simulink subsystem "MultibodySuspensionSSC"  (R2024a)
settings: Solver=VariableStepAuto  StartTime=0.0  StopTime=10.0  RelTol=1e-3
undefined symbols (not defined in the file): EnvGrvty, FrntRef, LAc, LAf, LAr, PlntVehDstCGFrntAxl, PlntVehDstCGRearAxl, PlntVehMass, PlntVehMultiBody, PlntVehMultiBodyGeom, RearRef, StrRodFL, StrRodFR, StrRodRL, StrRodRR, UAc, UAf, UAr, WheelFL, WheelFR, WheelRL, WheelRR, X, Y, Z
libraries: sm_lib x450, fl_lib x96, nesl_utility x64, sdl_lib x8
(part 10 of 17)

== system MultibodySuspensionSSC/SuspF/Linkage/Linkage R/DoubleWishbone/Upright ==
  note: Axle length still distance from
      | Wheel Center to Upright midpoint
  Axle : sm_lib/Body Elements/Cylindrical Solid  CylinderRadius=radius_stub_axle  CylinderRadiusUnits=m  CylinderLength=len_axle*2  CylinderLengthUnits=m  ExportEntireGeometry=off  InertiaType=PointMass  BasedOnType=Mass  Density=7000  DensityUnits=kg/m^3  Mass=0  MassUnits=kg  CenterOfMass=[0 0 0]  CenterOfMassUnits=m  MomentsOfInertia=[1 1 1]  MomentsOfInertiaUnits=kg*m^2  ProductsOfInertia=[0 0 0]  ProductsOfInertiaUnits=kg*m^2  GraphicType=FromGeometry  MarkerShape=Sphere  MarkerSize=10  GraphicVisPropType=SimpleVisualProperties  GraphicDiffuseColor=clr_stub_axle  GraphicOpacity=opc_stub_axle  GraphicSpecularColor=[0.5 0.5 0.5 1.0]  GraphicAmbientColor=[0.15 0.15 0.15 1.0]  GraphicEmissiveColor=[0.0 0.0 0.0 1.0]  GraphicShininess=75  DoExposeReferenceFrame=on  SerializedFrames=<Frames/>
      settings: LibrarySourceBlock=sm_car_4post_lib/Suspension and Steering/Linkage/Linkage R/DoubleWishbone/Upright/Axle
  Inertia CG : sm_lib/Body Elements/Inertia  InertiaType=PointMass  Mass=upr_mass  MassUnits=kg  CenterOfMass=[0 0 0]  CenterOfMassUnits=m  MomentsOfInertia=[1 1 1]  MomentsOfInertiaUnits=kg*m^2  ProductsOfInertia=[0 0 0]  ProductsOfInertiaUnits=kg*m^2  GraphicType=Marker  MarkerShape=Inertia  MarkerSize=20  GraphicVisPropType=SimpleVisualProperties  GraphicDiffuseColor=[0.5 0.5 0.5]  GraphicOpacity=0  GraphicSpecularColor=[0.5 0.5 0.5 1.0]  GraphicAmbientColor=[0.15 0.15 0.15 1.0]  GraphicEmissiveColor=[0.0 0.0 0.0 1.0]  GraphicShininess=75
      settings: LibrarySourceBlock=|
      | sm_car_4post_lib/Suspension and Steering/Linkage/Linkage R/DoubleWishbone/Upright/Inertia
      | CG
  Steering Arm : Subsystem  mask{hp_b=(hp_la_out+(35/300)*(hp_ua_out-hp_la_out)).*rhs_hp, hp_f=hp_upr_rod.*rhs_hp, Mass=0, clr_solid=clr_upr, opc_solid=opc_upr, rad_solid=radius_upr}
      mask prompts: hp_b "Hardpoint at B [xyz] (m)"; hp_f "Hardpoint at F [xyz] (m)"; Mass "Mass (kg)"; clr_solid "Color [RGB]"; opc_solid "Opacity (0-1)"; rad_solid "Radius (m)"
      settings: LibrarySourceBlock=sm_car_4post_lib/Suspension and Steering/Linkage/Linkage R/DoubleWishbone/Upright/Steering Arm
      mask TypeOptions Mass: Solid/Mass
      mask TypeOptions clr_solid: Solid/GraphicDiffuseColor
      mask TypeOptions opc_solid: Solid/GraphicOpacity
      mask TypeOptions rad_solid: Solid/CylinderRadius
      mask DialogControl cont_vis Prompt: Visualization
  Transform Align for Universal Joint : Subsystem  mask(Transform Align Axis Two Points){hp_b=(hp_la_out+0.5*(hp_ua_out-hp_la_out)).*rhs_hp, hp_t=hp_upr_rod.*rhs_hp, popup_f_axis=+Z}
      mask prompts: hp_b "Location of B [xyz] (m)"; hp_t "Target for Frame Axis [xyz] (m)"; popup_f_axis "Axis of F Frame to Aim at Target"
      mask help: Transforms a frame to aim a selected axis at a target point. Both points must be defined relative to the same reference frame.
      mask init: same as MultibodySuspensionSSC/SuspF/Linkage/Linkage L/DoubleWishbone/Hardpoints/Transform Align LAf LAr
      settings: LibrarySourceBlock=|
      | sm_car_4post_lib/Suspension and Steering/Linkage/Linkage R/DoubleWishbone/Upright/Transform
      | Align for
      | Universal
      | Joint
      mask TypeOptions popup_f_axis: +X | +Y | +Z | -X | -Y | -Z
  Transform Toe Camber : sm_lib/Frames and Transforms/Rigid Transform  RotationMethod=RotationSequence  FollAlignAxisA=+X  BaseAlignAxisA=+Y  FollAlignAxisB=+Y  BaseAlignAxisB=+Z  RotationStandardAxis=+Z  RotationAngle=0.0  RotationAngleUnits=deg  RotationArbitraryAxis=[0 0 1]  RotationSequenceAxes=FollowerAxes  RotationSequence=YXY  RotationSequenceAngles=[atoe -acamber 0].*rhs_upr  RotationSequenceAnglesUnits=deg  RotationMatrix=[1 0 0; 0 1 0; 0 0 1]  Quaternion=[1 0 0 0]  TranslationMethod=None  TranslationCartesianOffset=[0 0 0]  TranslationCartesianOffsetUnits=m  TranslationStandardAxis=+Z  TranslationStandardOffset=0  TranslationStandardOffsetUnits=m  TranslationROffset=0  TranslationROffsetUnits=m  TranslationThetaOffset=0  TranslationThetaOffsetUnits=deg  TranslationZOffset=0  TranslationZOffsetUnits=m
      settings: LibrarySourceBlock=|
      | sm_car_4post_lib/Suspension and Steering/Linkage/Linkage R/DoubleWishbone/Upright/Transform
      | Toe Camber
  Transform Upright CG : sm_lib/Frames and Transforms/Rigid Transform  RotationMethod=None  FollAlignAxisA=+X  BaseAlignAxisA=+Y  FollAlignAxisB=+Y  BaseAlignAxisB=+Z  RotationStandardAxis=+Z  RotationAngle=0.0  RotationAngleUnits=deg  RotationArbitraryAxis=[0 0 1]  RotationSequenceAxes=FollowerAxes  RotationSequence=XYX  RotationSequenceAngles=[0 0 0]  RotationSequenceAnglesUnits=deg  RotationMatrix=[1 0 0; 0 1 0; 0 0 1]  Quaternion=[1 0 0 0]  TranslationMethod=Cartesian  TranslationCartesianOffset=(hp_upr_cg-hp_la_out) .* [1, rhs_upr, 1]  TranslationCartesianOffsetUnits=m  TranslationStandardAxis=+Z  TranslationStandardOffset=0  TranslationStandardOffsetUnits=m  TranslationROffset=0  TranslationROffsetUnits=m  TranslationThetaOffset=0  TranslationThetaOffsetUnits=deg  TranslationZOffset=0  TranslationZOffsetUnits=m
      settings: LibrarySourceBlock=|
      | sm_car_4post_lib/Suspension and Steering/Linkage/Linkage R/DoubleWishbone/Upright/Transform
      | Upright CG
  Transform Upright Ctr : sm_lib/Frames and Transforms/Rigid Transform  RotationMethod=None  FollAlignAxisA=+X  BaseAlignAxisA=+Y  FollAlignAxisB=+Y  BaseAlignAxisB=+Z  RotationStandardAxis=+Z  RotationAngle=0.0  RotationAngleUnits=deg  RotationArbitraryAxis=[0 0 1]  RotationSequenceAxes=FollowerAxes  RotationSequence=XYX  RotationSequenceAngles=[0 0 0]  RotationSequenceAnglesUnits=deg  RotationMatrix=[1 0 0; 0 1 0; 0 0 1]  Quaternion=[1 0 0 0]  TranslationMethod=Cartesian  TranslationCartesianOffset=(35/300)*(hp_ua_out-hp_la_out).*rhs_hp  TranslationCartesianOffsetUnits=m  TranslationStandardAxis=+Z  TranslationStandardOffset=0  TranslationStandardOffsetUnits=m  TranslationROffset=0  TranslationROffsetUnits=m  TranslationThetaOffset=0  TranslationThetaOffsetUnits=deg  TranslationZOffset=0  TranslationZOffsetUnits=m
      settings: LibrarySourceBlock=|
      | sm_car_4post_lib/Suspension and Steering/Linkage/Linkage R/DoubleWishbone/Upright/Transform
      | Upright Ctr
  Transform Whl Ctr : sm_lib/Frames and Transforms/Rigid Transform  RotationMethod=AlignedAxes  FollAlignAxisA=+Z  BaseAlignAxisA=+Y  FollAlignAxisB=+X  BaseAlignAxisB=+X  RotationStandardAxis=+Z  RotationAngle=0.0  RotationAngleUnits=deg  RotationArbitraryAxis=[0 0 1]  RotationSequenceAxes=FollowerAxes  RotationSequence=XYX  RotationSequenceAngles=[0 0 0]  RotationSequenceAnglesUnits=deg  RotationMatrix=[1 0 0; 0 1 0; 0 0 1]  Quaternion=[1 0 0 0]  TranslationMethod=Cartesian  TranslationCartesianOffset=(hp_upr_wc-hp_la_out) .* rhs_hp  TranslationCartesianOffsetUnits=m  TranslationStandardAxis=+Z  TranslationStandardOffset=0  TranslationStandardOffsetUnits=m  TranslationROffset=0  TranslationROffsetUnits=m  TranslationThetaOffset=0  TranslationThetaOffsetUnits=deg  TranslationZOffset=0  TranslationZOffsetUnits=m
      settings: LibrarySourceBlock=|
      | sm_car_4post_lib/Suspension and Steering/Linkage/Linkage R/DoubleWishbone/Upright/Transform
      | Whl Ctr
  Upright : Subsystem  mask{hp_b=hp_la_out.*rhs_hp, hp_f=hp_ua_out.*rhs_hp, Mass=0, clr_solid=clr_upr, opc_solid=opc_upr, rad_solid=radius_upr}
      mask prompts: hp_b "Hardpoint at B [xyz] (m)"; hp_f "Hardpoint at F [xyz] (m)"; Mass "Mass (kg)"; clr_solid "Color [RGB]"; opc_solid "Opacity (0-1)"; rad_solid "Radius (m)"
      settings: LibrarySourceBlock=sm_car_4post_lib/Suspension and Steering/Linkage/Linkage R/DoubleWishbone/Upright/Upright
      mask TypeOptions Mass: Solid/Mass
      mask TypeOptions clr_solid: Solid/GraphicDiffuseColor
      mask TypeOptions opc_solid: Solid/GraphicOpacity
      mask TypeOptions rad_solid: Solid/CylinderRadius
      mask DialogControl cont_vis Prompt: Visualization
  Vis Upright LA : sm_lib/Body Elements/Spherical Solid  SphereRadius=size_conn_upr  SphereRadiusUnits=m  ExportEntireGeometry=off  InertiaType=PointMass  BasedOnType=Density  Density=0  DensityUnits=kg/m^3  Mass=0  MassUnits=kg  CenterOfMass=[0 0 0]  CenterOfMassUnits=m  MomentsOfInertia=[1 1 1]  MomentsOfInertiaUnits=kg*m^2  ProductsOfInertia=[0 0 0]  ProductsOfInertiaUnits=kg*m^2  GraphicType=FromGeometry  MarkerShape=Sphere  MarkerSize=10  GraphicVisPropType=SimpleVisualProperties  GraphicDiffuseColor=clr_conn_upr  GraphicOpacity=opc_conn_upr  GraphicSpecularColor=[0.5 0.5 0.5 1.0]  GraphicAmbientColor=[0.15 0.15 0.15 1.0]  GraphicEmissiveColor=[0.0 0.0 0.0 1.0]  GraphicShininess=75  DoExposeReferenceFrame=on  SerializedFrames=<Frames/>
      settings: LibrarySourceBlock=sm_car_4post_lib/Suspension and Steering/Linkage/Linkage R/DoubleWishbone/Upright/Vis Upright LA
  Vis Upright UA : sm_lib/Body Elements/Spherical Solid  SphereRadius=size_conn_upr  SphereRadiusUnits=m  ExportEntireGeometry=off  InertiaType=PointMass  BasedOnType=Density  Density=0  DensityUnits=kg/m^3  Mass=0  MassUnits=kg  CenterOfMass=[0 0 0]  CenterOfMassUnits=m  MomentsOfInertia=[1 1 1]  MomentsOfInertiaUnits=kg*m^2  ProductsOfInertia=[0 0 0]  ProductsOfInertiaUnits=kg*m^2  GraphicType=FromGeometry  MarkerShape=Sphere  MarkerSize=10  GraphicVisPropType=SimpleVisualProperties  GraphicDiffuseColor=clr_conn_upr  GraphicOpacity=opc_conn_upr  GraphicSpecularColor=[0.5 0.5 0.5 1.0]  GraphicAmbientColor=[0.15 0.15 0.15 1.0]  GraphicEmissiveColor=[0.0 0.0 0.0 1.0]  GraphicShininess=75  DoExposeReferenceFrame=on  SerializedFrames=<Frames/>
      settings: LibrarySourceBlock=sm_car_4post_lib/Suspension and Steering/Linkage/Linkage R/DoubleWishbone/Upright/Vis Upright UA
  Vis Wheel Center : sm_lib/Body Elements/Spherical Solid  SphereRadius=size_conn_upr  SphereRadiusUnits=m  ExportEntireGeometry=off  InertiaType=PointMass  BasedOnType=Density  Density=0  DensityUnits=kg/m^3  Mass=0  MassUnits=kg  CenterOfMass=[0 0 0]  CenterOfMassUnits=m  MomentsOfInertia=[1 1 1]  MomentsOfInertiaUnits=kg*m^2  ProductsOfInertia=[0 0 0]  ProductsOfInertiaUnits=kg*m^2  GraphicType=FromGeometry  MarkerShape=Sphere  MarkerSize=10  GraphicVisPropType=SimpleVisualProperties  GraphicDiffuseColor=clr_conn_upr  GraphicOpacity=opc_conn_upr  GraphicSpecularColor=[0.5 0.5 0.5 1.0]  GraphicAmbientColor=[0.15 0.15 0.15 1.0]  GraphicEmissiveColor=[0.0 0.0 0.0 1.0]  GraphicShininess=75  DoExposeReferenceFrame=on  SerializedFrames=<Frames/>
      settings: LibrarySourceBlock=sm_car_4post_lib/Suspension and Steering/Linkage/Linkage R/DoubleWishbone/Upright/Vis Wheel Center
  Tyre : PMIOPort  Side=Left
  Rod : PMIOPort  Port=2  Side=Right
  UA : PMIOPort  Port=3  Side=Right
  LA : PMIOPort  Port=4  Side=Right
  connections:
  Tyre/RConn1 -- Transform Toe Camber/RConn1 -- Vis Wheel Center/RConn1 -- Axle/RConn1
  LA/RConn1 -- Transform Whl Ctr/LConn1 -- Upright/LConn1 -- Transform Upright Ctr/LConn1 -- Transform Upright CG/LConn1 -- Vis Upright LA/RConn1
  Vis Upright UA/RConn1 -- Upright/RConn1 -- UA/RConn1
  Transform Upright CG/RConn1 -- Inertia CG/RConn1
  Steering Arm/LConn1 -- Transform Upright Ctr/RConn1
  Rod/RConn1 -- Transform Align for Universal Joint/RConn1
  Transform Align for Universal Joint/LConn1 -- Steering Arm/RConn1
  Transform Toe Camber/LConn1 -- Transform Whl Ctr/RConn1

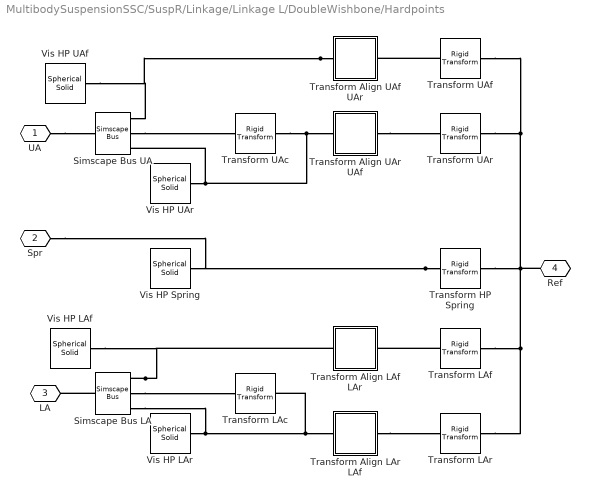
== system MultibodySuspensionSSC/SuspR/Linkage/Linkage L/DoubleWishbone/Hardpoints ==
  Simscape Bus LA : SimscapeBus  HierarchyStrings=LAf;LAc;LAr
  Simscape Bus UA : SimscapeBus  HierarchyStrings=UAf;UAc;UAr
  Transform Align LAf LAr : Subsystem  mask(Transform Align Axis Two Points){hp_b=hp_in_f_la.*rhs_hp, hp_t=hp_in_r_la.*rhs_hp, popup_f_axis=-Z}
      mask prompts: hp_b "Location of B [xyz] (m)"; hp_t "Target for Frame Axis [xyz] (m)"; popup_f_axis "Axis of F Frame to Aim at Target"
      mask help: Transforms a frame to aim a selected axis at a target point. Both points must be defined relative to the same reference frame.
      mask init: same as MultibodySuspensionSSC/SuspF/Linkage/Linkage L/DoubleWishbone/Hardpoints/Transform Align LAf LAr
      settings: LibrarySourceBlock=|
      | sm_car_4post_lib/Suspension and Steering/Linkage/Linkage L/DoubleWishbone/Hardpoints/Transform
      | Align LAf LAr
      mask TypeOptions popup_f_axis: +X | +Y | +Z | -X | -Y | -Z
  Transform Align LAr LAf : Subsystem  mask(Transform Align Axis Two Points){hp_b=hp_in_r_la.*rhs_hp, hp_t=hp_in_f_la.*rhs_hp, popup_f_axis=+Z}
      mask prompts: hp_b "Location of B [xyz] (m)"; hp_t "Target for Frame Axis [xyz] (m)"; popup_f_axis "Axis of F Frame to Aim at Target"
      mask help: Transforms a frame to aim a selected axis at a target point. Both points must be defined relative to the same reference frame.
      mask init: same as MultibodySuspensionSSC/SuspF/Linkage/Linkage L/DoubleWishbone/Hardpoints/Transform Align LAf LAr
      settings: LibrarySourceBlock=|
      | sm_car_4post_lib/Suspension and Steering/Linkage/Linkage L/DoubleWishbone/Hardpoints/Transform
      | Align LAr LAf
      mask TypeOptions popup_f_axis: +X | +Y | +Z | -X | -Y | -Z
  Transform Align UAf UAr : Subsystem  mask(Transform Align Axis Two Points){hp_b=hp_in_f_ua.*rhs_hp, hp_t=hp_in_r_ua.*rhs_hp, popup_f_axis=-Z}
      mask prompts: hp_b "Location of B [xyz] (m)"; hp_t "Target for Frame Axis [xyz] (m)"; popup_f_axis "Axis of F Frame to Aim at Target"
      mask help: Transforms a frame to aim a selected axis at a target point. Both points must be defined relative to the same reference frame.
      mask init: same as MultibodySuspensionSSC/SuspF/Linkage/Linkage L/DoubleWishbone/Hardpoints/Transform Align LAf LAr
      settings: LibrarySourceBlock=|
      | sm_car_4post_lib/Suspension and Steering/Linkage/Linkage L/DoubleWishbone/Hardpoints/Transform
      | Align UAf UAr
      mask TypeOptions popup_f_axis: +X | +Y | +Z | -X | -Y | -Z
  Transform Align UAr UAf : Subsystem  mask(Transform Align Axis Two Points){hp_b=hp_in_r_ua.*rhs_hp, hp_t=hp_in_f_ua.*rhs_hp, popup_f_axis=+Z}
      mask prompts: hp_b "Location of B [xyz] (m)"; hp_t "Target for Frame Axis [xyz] (m)"; popup_f_axis "Axis of F Frame to Aim at Target"
      mask help: Transforms a frame to aim a selected axis at a target point. Both points must be defined relative to the same reference frame.
      mask init: same as MultibodySuspensionSSC/SuspF/Linkage/Linkage L/DoubleWishbone/Hardpoints/Transform Align LAf LAr
      settings: LibrarySourceBlock=|
      | sm_car_4post_lib/Suspension and Steering/Linkage/Linkage L/DoubleWishbone/Hardpoints/Transform
      | Align UAr UAf
      mask TypeOptions popup_f_axis: +X | +Y | +Z | -X | -Y | -Z
  Transform HP Spring : sm_lib/Frames and Transforms/Rigid Transform  RotationMethod=None  FollAlignAxisA=+X  BaseAlignAxisA=+Y  FollAlignAxisB=+Y  BaseAlignAxisB=+Z  RotationStandardAxis=+Z  RotationAngle=0.0  RotationAngleUnits=deg  RotationArbitraryAxis=[0 0 1]  RotationSequenceAxes=FollowerAxes  RotationSequence=XYX  RotationSequenceAngles=[0 0 0]  RotationSequenceAnglesUnits=deg  RotationMatrix=[1 0 0; 0 1 0; 0 0 1]  Quaternion=[1 0 0 0]  TranslationMethod=Cartesian  TranslationCartesianOffset=hp_spr_top.*rhs_hp  TranslationCartesianOffsetUnits=m  TranslationStandardAxis=+Z  TranslationStandardOffset=0  TranslationStandardOffsetUnits=m  TranslationROffset=0  TranslationROffsetUnits=m  TranslationThetaOffset=0  TranslationThetaOffsetUnits=deg  TranslationZOffset=0  TranslationZOffsetUnits=m
      settings: LibrarySourceBlock=sm_car_4post_lib/Suspension and Steering/Linkage/Linkage L/DoubleWishbone/Hardpoints/Transform HP Spring
  Transform LAc : sm_lib/Frames and Transforms/Rigid Transform  RotationMethod=None  FollAlignAxisA=+X  BaseAlignAxisA=+Y  FollAlignAxisB=+Y  BaseAlignAxisB=+Z  RotationStandardAxis=+Z  RotationAngle=0  RotationAngleUnits=deg  RotationArbitraryAxis=[0 0 1]  RotationSequenceAxes=FollowerAxes  RotationSequence=XYX  RotationSequenceAngles=[0 0 0]  RotationSequenceAnglesUnits=deg  RotationMatrix=[0 0 -1;0 1 0;1 0 0]  Quaternion=[1 0 0 0]  TranslationMethod=StandardAxis  TranslationCartesianOffset=[0 0 0]  TranslationCartesianOffsetUnits=m  TranslationStandardAxis=+Z  TranslationStandardOffset=norm(hp_in_f_la-hp_in_r_la)/2  TranslationStandardOffsetUnits=m  TranslationROffset=0  TranslationROffsetUnits=m  TranslationThetaOffset=0  TranslationThetaOffsetUnits=deg  TranslationZOffset=0  TranslationZOffsetUnits=m
      settings: LibrarySourceBlock=sm_car_4post_lib/Suspension and Steering/Linkage/Linkage L/DoubleWishbone/Hardpoints/Transform LAc
  Transform LAf : sm_lib/Frames and Transforms/Rigid Transform  RotationMethod=None  FollAlignAxisA=+X  BaseAlignAxisA=+Y  FollAlignAxisB=+Y  BaseAlignAxisB=+Z  RotationStandardAxis=+Z  RotationAngle=0.0  RotationAngleUnits=deg  RotationArbitraryAxis=[0 0 1]  RotationSequenceAxes=FollowerAxes  RotationSequence=XYX  RotationSequenceAngles=[0 0 0]  RotationSequenceAnglesUnits=deg  RotationMatrix=[1 0 0; 0 1 0; 0 0 1]  Quaternion=[1 0 0 0]  TranslationMethod=Cartesian  TranslationCartesianOffset=hp_in_f_la.*rhs_hp  TranslationCartesianOffsetUnits=m  TranslationStandardAxis=+Z  TranslationStandardOffset=0  TranslationStandardOffsetUnits=m  TranslationROffset=0  TranslationROffsetUnits=m  TranslationThetaOffset=0  TranslationThetaOffsetUnits=deg  TranslationZOffset=0  TranslationZOffsetUnits=m
      settings: LibrarySourceBlock=sm_car_4post_lib/Suspension and Steering/Linkage/Linkage L/DoubleWishbone/Hardpoints/Transform LAf
  Transform LAr : sm_lib/Frames and Transforms/Rigid Transform  RotationMethod=None  FollAlignAxisA=+X  BaseAlignAxisA=+Y  FollAlignAxisB=+Y  BaseAlignAxisB=+Z  RotationStandardAxis=+Z  RotationAngle=0.0  RotationAngleUnits=deg  RotationArbitraryAxis=[0 0 1]  RotationSequenceAxes=FollowerAxes  RotationSequence=XYX  RotationSequenceAngles=[0 0 0]  RotationSequenceAnglesUnits=deg  RotationMatrix=[1 0 0; 0 1 0; 0 0 1]  Quaternion=[1 0 0 0]  TranslationMethod=Cartesian  TranslationCartesianOffset=hp_in_r_la.*rhs_hp  TranslationCartesianOffsetUnits=m  TranslationStandardAxis=+Z  TranslationStandardOffset=0  TranslationStandardOffsetUnits=m  TranslationROffset=0  TranslationROffsetUnits=m  TranslationThetaOffset=0  TranslationThetaOffsetUnits=deg  TranslationZOffset=0  TranslationZOffsetUnits=m
      settings: LibrarySourceBlock=sm_car_4post_lib/Suspension and Steering/Linkage/Linkage L/DoubleWishbone/Hardpoints/Transform LAr
  Transform UAc : sm_lib/Frames and Transforms/Rigid Transform  RotationMethod=None  FollAlignAxisA=+X  BaseAlignAxisA=+Y  FollAlignAxisB=+Y  BaseAlignAxisB=+Z  RotationStandardAxis=+Z  RotationAngle=0  RotationAngleUnits=deg  RotationArbitraryAxis=[0 0 1]  RotationSequenceAxes=FollowerAxes  RotationSequence=XYX  RotationSequenceAngles=[0 0 0]  RotationSequenceAnglesUnits=deg  RotationMatrix=[0 0 -1;0 1 0;1 0 0]  Quaternion=[1 0 0 0]  TranslationMethod=StandardAxis  TranslationCartesianOffset=[0 0 0]  TranslationCartesianOffsetUnits=m  TranslationStandardAxis=+Z  TranslationStandardOffset=norm(hp_in_f_ua - hp_in_r_ua)/2  TranslationStandardOffsetUnits=m  TranslationROffset=0  TranslationROffsetUnits=m  TranslationThetaOffset=0  TranslationThetaOffsetUnits=deg  TranslationZOffset=0  TranslationZOffsetUnits=m
      settings: LibrarySourceBlock=sm_car_4post_lib/Suspension and Steering/Linkage/Linkage L/DoubleWishbone/Hardpoints/Transform UAc
  Transform UAf : sm_lib/Frames and Transforms/Rigid Transform  RotationMethod=None  FollAlignAxisA=+X  BaseAlignAxisA=+Y  FollAlignAxisB=+Y  BaseAlignAxisB=+Z  RotationStandardAxis=+Z  RotationAngle=0.0  RotationAngleUnits=deg  RotationArbitraryAxis=[0 0 1]  RotationSequenceAxes=FollowerAxes  RotationSequence=XYX  RotationSequenceAngles=[0 0 0]  RotationSequenceAnglesUnits=deg  RotationMatrix=[1 0 0; 0 1 0; 0 0 1]  Quaternion=[1 0 0 0]  TranslationMethod=Cartesian  TranslationCartesianOffset=hp_in_f_ua.*rhs_hp  TranslationCartesianOffsetUnits=m  TranslationStandardAxis=+Z  TranslationStandardOffset=0  TranslationStandardOffsetUnits=m  TranslationROffset=0  TranslationROffsetUnits=m  TranslationThetaOffset=0  TranslationThetaOffsetUnits=deg  TranslationZOffset=0  TranslationZOffsetUnits=m
      settings: LibrarySourceBlock=sm_car_4post_lib/Suspension and Steering/Linkage/Linkage L/DoubleWishbone/Hardpoints/Transform UAf
  Transform UAr : sm_lib/Frames and Transforms/Rigid Transform  RotationMethod=None  FollAlignAxisA=+X  BaseAlignAxisA=+Y  FollAlignAxisB=+Y  BaseAlignAxisB=+Z  RotationStandardAxis=+Z  RotationAngle=0.0  RotationAngleUnits=deg  RotationArbitraryAxis=[0 0 1]  RotationSequenceAxes=FollowerAxes  RotationSequence=XYX  RotationSequenceAngles=[0 0 0]  RotationSequenceAnglesUnits=deg  RotationMatrix=[1 0 0; 0 1 0; 0 0 1]  Quaternion=[1 0 0 0]  TranslationMethod=Cartesian  TranslationCartesianOffset=hp_in_r_ua.*rhs_hp  TranslationCartesianOffsetUnits=m  TranslationStandardAxis=+Z  TranslationStandardOffset=0  TranslationStandardOffsetUnits=m  TranslationROffset=0  TranslationROffsetUnits=m  TranslationThetaOffset=0  TranslationThetaOffsetUnits=deg  TranslationZOffset=0  TranslationZOffsetUnits=m
      settings: LibrarySourceBlock=sm_car_4post_lib/Suspension and Steering/Linkage/Linkage L/DoubleWishbone/Hardpoints/Transform UAr
  Vis HP LAf : sm_lib/Body Elements/Spherical Solid  SphereRadius=size_hp  SphereRadiusUnits=m  ExportEntireGeometry=off  InertiaType=CalculateFromGeometry  BasedOnType=Density  Density=0  DensityUnits=kg/m^3  Mass=1  MassUnits=kg  CenterOfMass=[0 0 0]  CenterOfMassUnits=m  MomentsOfInertia=[1 1 1]  MomentsOfInertiaUnits=kg*m^2  ProductsOfInertia=[0 0 0]  ProductsOfInertiaUnits=kg*m^2  GraphicType=FromGeometry  MarkerShape=Sphere  MarkerSize=10  GraphicVisPropType=SimpleVisualProperties  GraphicDiffuseColor=clr_hp  GraphicOpacity=opc_hp  GraphicSpecularColor=[0.5 0.5 0.5 1.0]  GraphicAmbientColor=[0.15 0.15 0.15 1.0]  GraphicEmissiveColor=[0.0 0.0 0.0 1.0]  GraphicShininess=75  DoExposeReferenceFrame=on  SerializedFrames=<Frames/>
      settings: LibrarySourceBlock=sm_car_4post_lib/Suspension and Steering/Linkage/Linkage L/DoubleWishbone/Hardpoints/Vis HP LAf
  Vis HP LAr : sm_lib/Body Elements/Spherical Solid  SphereRadius=size_hp  SphereRadiusUnits=m  ExportEntireGeometry=off  InertiaType=CalculateFromGeometry  BasedOnType=Density  Density=0  DensityUnits=kg/m^3  Mass=1  MassUnits=kg  CenterOfMass=[0 0 0]  CenterOfMassUnits=m  MomentsOfInertia=[1 1 1]  MomentsOfInertiaUnits=kg*m^2  ProductsOfInertia=[0 0 0]  ProductsOfInertiaUnits=kg*m^2  GraphicType=FromGeometry  MarkerShape=Sphere  MarkerSize=10  GraphicVisPropType=SimpleVisualProperties  GraphicDiffuseColor=clr_hp  GraphicOpacity=opc_hp  GraphicSpecularColor=[0.5 0.5 0.5 1.0]  GraphicAmbientColor=[0.15 0.15 0.15 1.0]  GraphicEmissiveColor=[0.0 0.0 0.0 1.0]  GraphicShininess=75  DoExposeReferenceFrame=on  SerializedFrames=<Frames/>
      settings: LibrarySourceBlock=sm_car_4post_lib/Suspension and Steering/Linkage/Linkage L/DoubleWishbone/Hardpoints/Vis HP LAr
  Vis HP Spring : sm_lib/Body Elements/Spherical Solid  SphereRadius=size_hp  SphereRadiusUnits=m  ExportEntireGeometry=off  InertiaType=CalculateFromGeometry  BasedOnType=Density  Density=0  DensityUnits=kg/m^3  Mass=1  MassUnits=kg  CenterOfMass=[0 0 0]  CenterOfMassUnits=m  MomentsOfInertia=[1 1 1]  MomentsOfInertiaUnits=kg*m^2  ProductsOfInertia=[0 0 0]  ProductsOfInertiaUnits=kg*m^2  GraphicType=FromGeometry  MarkerShape=Sphere  MarkerSize=10  GraphicVisPropType=SimpleVisualProperties  GraphicDiffuseColor=clr_hp  GraphicOpacity=opc_hp  GraphicSpecularColor=[0.5 0.5 0.5 1.0]  GraphicAmbientColor=[0.15 0.15 0.15 1.0]  GraphicEmissiveColor=[0.0 0.0 0.0 1.0]  GraphicShininess=75  DoExposeReferenceFrame=on  SerializedFrames=<Frames/>
      settings: LibrarySourceBlock=sm_car_4post_lib/Suspension and Steering/Linkage/Linkage L/DoubleWishbone/Hardpoints/Vis HP Spring
  Vis HP UAf : sm_lib/Body Elements/Spherical Solid  SphereRadius=size_hp  SphereRadiusUnits=m  ExportEntireGeometry=off  InertiaType=CalculateFromGeometry  BasedOnType=Density  Density=0  DensityUnits=kg/m^3  Mass=1  MassUnits=kg  CenterOfMass=[0 0 0]  CenterOfMassUnits=m  MomentsOfInertia=[1 1 1]  MomentsOfInertiaUnits=kg*m^2  ProductsOfInertia=[0 0 0]  ProductsOfInertiaUnits=kg*m^2  GraphicType=FromGeometry  MarkerShape=Sphere  MarkerSize=10  GraphicVisPropType=SimpleVisualProperties  GraphicDiffuseColor=clr_hp  GraphicOpacity=opc_hp  GraphicSpecularColor=[0.5 0.5 0.5 1.0]  GraphicAmbientColor=[0.15 0.15 0.15 1.0]  GraphicEmissiveColor=[0.0 0.0 0.0 1.0]  GraphicShininess=75  DoExposeReferenceFrame=on  SerializedFrames=<Frames/>
      settings: LibrarySourceBlock=sm_car_4post_lib/Suspension and Steering/Linkage/Linkage L/DoubleWishbone/Hardpoints/Vis HP UAf
  Vis HP UAr : sm_lib/Body Elements/Spherical Solid  SphereRadius=size_hp  SphereRadiusUnits=m  ExportEntireGeometry=off  InertiaType=CalculateFromGeometry  BasedOnType=Density  Density=0  DensityUnits=kg/m^3  Mass=1  MassUnits=kg  CenterOfMass=[0 0 0]  CenterOfMassUnits=m  MomentsOfInertia=[1 1 1]  MomentsOfInertiaUnits=kg*m^2  ProductsOfInertia=[0 0 0]  ProductsOfInertiaUnits=kg*m^2  GraphicType=FromGeometry  MarkerShape=Sphere  MarkerSize=10  GraphicVisPropType=SimpleVisualProperties  GraphicDiffuseColor=clr_hp  GraphicOpacity=opc_hp  GraphicSpecularColor=[0.5 0.5 0.5 1.0]  GraphicAmbientColor=[0.15 0.15 0.15 1.0]  GraphicEmissiveColor=[0.0 0.0 0.0 1.0]  GraphicShininess=75  DoExposeReferenceFrame=on  SerializedFrames=<Frames/>
      settings: LibrarySourceBlock=sm_car_4post_lib/Suspension and Steering/Linkage/Linkage L/DoubleWishbone/Hardpoints/Vis HP UAr
  UA : PMIOPort  Side=Left
  Spr : PMIOPort  Port=2  Side=Left
  LA : PMIOPort  Port=3  Side=Left
  Ref : PMIOPort  Port=4  Side=Right
  connections:
  Simscape Bus LA/RConn1 -- LA/RConn1
  Simscape Bus LA/LConn2 -- Transform LAc/RConn1
  UA/RConn1 -- Simscape Bus UA/RConn1
  Simscape Bus UA/LConn2 -- Transform UAc/RConn1
  Transform LAr/LConn1 -- Transform LAf/LConn1 -- Transform HP Spring/LConn1 -- Transform UAr/LConn1 -- Transform UAf/LConn1 -- Ref/RConn1
  Simscape Bus LA/LConn1 -- Transform Align LAf LAr/RConn1 -- Vis HP LAf/RConn1
  Simscape Bus LA/LConn3 -- Transform LAc/LConn1 -- Transform Align LAr LAf/RConn1 -- Vis HP LAr/RConn1
  Transform Align UAf UAr/RConn1 -- Vis HP UAf/RConn1 -- Simscape Bus UA/LConn1
  Transform HP Spring/RConn1 -- Spr/RConn1 -- Vis HP Spring/RConn1
  Transform UAf/RConn1 -- Transform Align UAf UAr/LConn1
  Transform Align UAr UAf/LConn1 -- Transform UAr/RConn1
  Transform UAc/LConn1 -- Simscape Bus UA/LConn3 -- Vis HP UAr/RConn1 -- Transform Align UAr UAf/RConn1
  Transform Align LAr LAf/LConn1 -- Transform LAr/RConn1
  Transform LAf/RConn1 -- Transform Align LAf LAr/LConn1

== system MultibodySuspensionSSC/SuspR/Linkage/Linkage L/DoubleWishbone/Lower Arm ==
  Arm F : Subsystem  mask{hp_b=hp_in_f.*rhs_hp, hp_f=hp_out.*rhs_hp, Mass=la_mass/2, clr_solid=clr_la, opc_solid=opc_la, rad_solid=radius_la}
      mask prompts: hp_b "Hardpoint at B [xyz] (m)"; hp_f "Hardpoint at F [xyz] (m)"; Mass "Mass (kg)"; clr_solid "Color [RGB]"; opc_solid "Opacity (0-1)"; rad_solid "Radius (m)"
      settings: LibrarySourceBlock=sm_car_4post_lib/Suspension and Steering/Linkage/Linkage L/DoubleWishbone/Lower Arm/Arm F
      mask TypeOptions Mass: Solid/Mass
      mask TypeOptions clr_solid: Solid/GraphicDiffuseColor
      mask TypeOptions opc_solid: Solid/GraphicOpacity
      mask TypeOptions rad_solid: Solid/CylinderRadius
      mask DialogControl cont_vis Prompt: Visualization
  Arm R : Subsystem  mask{hp_b=hp_in_r.*rhs_hp, hp_f=hp_out.*rhs_hp, Mass=la_mass/2, clr_solid=clr_la, opc_solid=opc_la, rad_solid=radius_la}
      mask prompts: hp_b "Hardpoint at B [xyz] (m)"; hp_f "Hardpoint at F [xyz] (m)"; Mass "Mass (kg)"; clr_solid "Color [RGB]"; opc_solid "Opacity (0-1)"; rad_solid "Radius (m)"
      settings: LibrarySourceBlock=sm_car_4post_lib/Suspension and Steering/Linkage/Linkage L/DoubleWishbone/Lower Arm/Arm R
      mask TypeOptions Mass: Solid/Mass
      mask TypeOptions clr_solid: Solid/GraphicDiffuseColor
      mask TypeOptions opc_solid: Solid/GraphicOpacity
      mask TypeOptions rad_solid: Solid/CylinderRadius
      mask DialogControl cont_vis Prompt: Visualization
  Arm Spring : Subsystem  mask{hp_b=hp_spr.*rhs_hp, hp_f=hp_out.*rhs_hp, Mass=0, clr_solid=clr_la, opc_solid=opc_la, rad_solid=radius_la}
      mask prompts: hp_b "Hardpoint at B [xyz] (m)"; hp_f "Hardpoint at F [xyz] (m)"; Mass "Mass (kg)"; clr_solid "Color [RGB]"; opc_solid "Opacity (0-1)"; rad_solid "Radius (m)"
      settings: LibrarySourceBlock=sm_car_4post_lib/Suspension and Steering/Linkage/Linkage L/DoubleWishbone/Lower Arm/Arm Spring
      mask TypeOptions Mass: Solid/Mass
      mask TypeOptions clr_solid: Solid/GraphicDiffuseColor
      mask TypeOptions opc_solid: Solid/GraphicOpacity
      mask TypeOptions rad_solid: Solid/CylinderRadius
      mask DialogControl cont_vis Prompt: Visualization
  Simscape Bus HP : SimscapeBus  HierarchyStrings=LAf;LAc;LAr
  Transform Align UAf UAr : Subsystem  mask(Transform Align Axis Two Points){hp_b=hp_in_r.*rhs_hp, hp_t=hp_in_f.*rhs_hp, popup_f_axis=+Z}
      mask prompts: hp_b "Location of B [xyz] (m)"; hp_t "Target for Frame Axis [xyz] (m)"; popup_f_axis "Axis of F Frame to Aim at Target"
      mask help: Transforms a frame to aim a selected axis at a target point. Both points must be defined relative to the same reference frame.
      mask init: same as MultibodySuspensionSSC/SuspF/Linkage/Linkage L/DoubleWishbone/Hardpoints/Transform Align LAf LAr
      settings: LibrarySourceBlock=|
      | sm_car_4post_lib/Suspension and Steering/Linkage/Linkage L/DoubleWishbone/Lower Arm/Transform
      | Align UAf UAr
      mask TypeOptions popup_f_axis: +X | +Y | +Z | -X | -Y | -Z
  Transform Align UAr UAf : Subsystem  mask(Transform Align Axis Two Points){hp_b=hp_in_r.*rhs_hp, hp_t=hp_in_f.*rhs_hp, popup_f_axis=+Z}
      mask prompts: hp_b "Location of B [xyz] (m)"; hp_t "Target for Frame Axis [xyz] (m)"; popup_f_axis "Axis of F Frame to Aim at Target"
      mask help: Transforms a frame to aim a selected axis at a target point. Both points must be defined relative to the same reference frame.
      mask init: same as MultibodySuspensionSSC/SuspF/Linkage/Linkage L/DoubleWishbone/Hardpoints/Transform Align LAf LAr
      settings: LibrarySourceBlock=|
      | sm_car_4post_lib/Suspension and Steering/Linkage/Linkage L/DoubleWishbone/Lower Arm/Transform
      | Align UAr UAf
      mask TypeOptions popup_f_axis: +X | +Y | +Z | -X | -Y | -Z
  Transform Inboard FR Ctr : sm_lib/Frames and Transforms/Rigid Transform  RotationMethod=None  FollAlignAxisA=+X  BaseAlignAxisA=+Y  FollAlignAxisB=+Y  BaseAlignAxisB=+Z  RotationStandardAxis=+Z  RotationAngle=0.0  RotationAngleUnits=deg  RotationArbitraryAxis=[0 0 1]  RotationSequenceAxes=FollowerAxes  RotationSequence=XYX  RotationSequenceAngles=[0 0 0]  RotationSequenceAnglesUnits=deg  RotationMatrix=[1 0 0; 0 1 0; 0 0 1]  Quaternion=[1 0 0 0]  TranslationMethod=StandardAxis  TranslationCartesianOffset=[0 0 0]  TranslationCartesianOffsetUnits=m  TranslationStandardAxis=+Z  TranslationStandardOffset=norm(hp_in_f-hp_in_r)/2  TranslationStandardOffsetUnits=m  TranslationROffset=0  TranslationROffsetUnits=m  TranslationThetaOffset=0  TranslationThetaOffsetUnits=deg  TranslationZOffset=0  TranslationZOffsetUnits=m
      settings: LibrarySourceBlock=|
      | sm_car_4post_lib/Suspension and Steering/Linkage/Linkage L/DoubleWishbone/Lower Arm/Transform
      | Inboard
      | FR Ctr
  HP : PMIOPort  Side=Right
  Spr : PMIOPort  Port=2  Side=Left
  Upr : PMIOPort  Port=3  Side=Left
  connections:
  Transform Align UAr UAf/RConn1 -- Simscape Bus HP/LConn3 -- Transform Inboard FR Ctr/LConn1
  Transform Inboard FR Ctr/RConn1 -- Simscape Bus HP/LConn2
  Simscape Bus HP/RConn1 -- HP/RConn1
  Arm Spring/LConn1 -- Spr/RConn1
  Arm F/RConn1 -- Arm R/RConn1 -- Upr/RConn1 -- Arm Spring/RConn1
  Transform Align UAr UAf/LConn1 -- Arm R/LConn1
  Transform Align UAf UAr/LConn1 -- Arm F/LConn1
  Transform Align UAf UAr/RConn1 -- Simscape Bus HP/LConn1

== system MultibodySuspensionSSC/SuspR/Linkage/Linkage L/DoubleWishbone/Primitive Gimbal ==
  Revolute X : sm_lib/Joints/Revolute Joint  JointMode=Normal  CompositeWrenchDir=FollowerOnBase  CompositeWrenchFrame=BaseFrame  SenseConstraintForce=off  SenseConstraintTorque=off  SenseTotalForce=off  SenseTotalTorque=off  PositionTargetSpecify=off  PositionTargetPriority=High  PositionTargetValue=0  PositionTargetValueUnits=deg  VelocityTargetSpecify=off  VelocityTargetPriority=High  VelocityTargetValue=0  VelocityTargetValueUnits=deg/s  EquilibriumPosition=0  EquilibriumPositionUnits=deg  SpringStiffness=0  SpringStiffnessUnits=N*m/deg  DampingCoefficient=0  DampingCoefficientUnits=N*m/(deg/s)  LowerLimitSpecify=off  LowerLimitBound=-90  LowerLimitBoundUnits=deg  LowerLimitStiffness=1e4  LowerLimitStiffnessUnits=N*m/deg  LowerLimitDamping=10  LowerLimitDampingUnits=N*m/(deg/s)  LowerLimitTransitionRegionWidth=0.1  LowerLimitTransitionRegionWidthUnits=deg  UpperLimitSpecify=off  UpperLimitBound=90  UpperLimitBoundUnits=deg  UpperLimitStiffness=1e4  UpperLimitStiffnessUnits=N*m/deg  UpperLimitDamping=10  UpperLimitDampingUnits=N*m/(deg/s)  UpperLimitTransitionRegionWidth=0.1  UpperLimitTransitionRegionWidthUnits=deg  TorqueActuationMode=NoTorque  MotionActuationMode=ComputedMotion  SensePosition=off  SenseVelocity=off  SenseAcceleration=off  SenseTorqueForce=off  SenseLowerLimitTorqueForce=off  SenseUpperLimitTorqueForce=off
  Revolute Y : sm_lib/Joints/Revolute Joint  JointMode=Normal  CompositeWrenchDir=FollowerOnBase  CompositeWrenchFrame=BaseFrame  SenseConstraintForce=off  SenseConstraintTorque=off  SenseTotalForce=off  SenseTotalTorque=off  PositionTargetSpecify=off  PositionTargetPriority=High  PositionTargetValue=0  PositionTargetValueUnits=deg  VelocityTargetSpecify=off  VelocityTargetPriority=High  VelocityTargetValue=0  VelocityTargetValueUnits=deg/s  EquilibriumPosition=0  EquilibriumPositionUnits=deg  SpringStiffness=0  SpringStiffnessUnits=N*m/deg  DampingCoefficient=0  DampingCoefficientUnits=N*m/(deg/s)  LowerLimitSpecify=off  LowerLimitBound=-90  LowerLimitBoundUnits=deg  LowerLimitStiffness=1e4  LowerLimitStiffnessUnits=N*m/deg  LowerLimitDamping=10  LowerLimitDampingUnits=N*m/(deg/s)  LowerLimitTransitionRegionWidth=0.1  LowerLimitTransitionRegionWidthUnits=deg  UpperLimitSpecify=off  UpperLimitBound=90  UpperLimitBoundUnits=deg  UpperLimitStiffness=1e4  UpperLimitStiffnessUnits=N*m/deg  UpperLimitDamping=10  UpperLimitDampingUnits=N*m/(deg/s)  UpperLimitTransitionRegionWidth=0.1  UpperLimitTransitionRegionWidthUnits=deg  TorqueActuationMode=NoTorque  MotionActuationMode=ComputedMotion  SensePosition=off  SenseVelocity=off  SenseAcceleration=off  SenseTorqueForce=off  SenseLowerLimitTorqueForce=off  SenseUpperLimitTorqueForce=off
  Revolute Z : sm_lib/Joints/Revolute Joint  JointMode=Normal  CompositeWrenchDir=FollowerOnBase  CompositeWrenchFrame=BaseFrame  SenseConstraintForce=off  SenseConstraintTorque=off  SenseTotalForce=off  SenseTotalTorque=off  PositionTargetSpecify=off  PositionTargetPriority=High  PositionTargetValue=0  PositionTargetValueUnits=deg  VelocityTargetSpecify=off  VelocityTargetPriority=High  VelocityTargetValue=0  VelocityTargetValueUnits=deg/s  EquilibriumPosition=0  EquilibriumPositionUnits=deg  SpringStiffness=0  SpringStiffnessUnits=N*m/deg  DampingCoefficient=0  DampingCoefficientUnits=N*m/(deg/s)  LowerLimitSpecify=off  LowerLimitBound=-90  LowerLimitBoundUnits=deg  LowerLimitStiffness=1e4  LowerLimitStiffnessUnits=N*m/deg  LowerLimitDamping=10  LowerLimitDampingUnits=N*m/(deg/s)  LowerLimitTransitionRegionWidth=0.1  LowerLimitTransitionRegionWidthUnits=deg  UpperLimitSpecify=off  UpperLimitBound=90  UpperLimitBoundUnits=deg  UpperLimitStiffness=1e4  UpperLimitStiffnessUnits=N*m/deg  UpperLimitDamping=10  UpperLimitDampingUnits=N*m/(deg/s)  UpperLimitTransitionRegionWidth=0.1  UpperLimitTransitionRegionWidthUnits=deg  TorqueActuationMode=NoTorque  MotionActuationMode=ComputedMotion  SensePosition=off  SenseVelocity=off  SenseAcceleration=off  SenseTorqueForce=off  SenseLowerLimitTorqueForce=off  SenseUpperLimitTorqueForce=off
  Transform Revolute X : sm_lib/Frames and Transforms/Rigid Transform  RotationMethod=AlignedAxes  FollAlignAxisA=+Z  BaseAlignAxisA=+X  FollAlignAxisB=+Y  BaseAlignAxisB=+Y  RotationStandardAxis=+Z  RotationAngle=0.0  RotationAngleUnits=deg  RotationArbitraryAxis=[0 0 1]  RotationSequenceAxes=FollowerAxes  RotationSequence=XYX  RotationSequenceAngles=[0 0 0]  RotationSequenceAnglesUnits=deg  RotationMatrix=[1 0 0; 0 1 0; 0 0 1]  Quaternion=[1 0 0 0]  TranslationMethod=None  TranslationCartesianOffset=[0 0 0]  TranslationCartesianOffsetUnits=m  TranslationStandardAxis=+Z  TranslationStandardOffset=0  TranslationStandardOffsetUnits=m  TranslationROffset=0  TranslationROffsetUnits=m  TranslationThetaOffset=0  TranslationThetaOffsetUnits=deg  TranslationZOffset=0  TranslationZOffsetUnits=m
  Transform Revolute Y : sm_lib/Frames and Transforms/Rigid Transform  RotationMethod=AlignedAxes  FollAlignAxisA=+Z  BaseAlignAxisA=+Y  FollAlignAxisB=+X  BaseAlignAxisB=+Z  RotationStandardAxis=+Z  RotationAngle=0.0  RotationAngleUnits=deg  RotationArbitraryAxis=[0 0 1]  RotationSequenceAxes=FollowerAxes  RotationSequence=XYX  RotationSequenceAngles=[0 0 0]  RotationSequenceAnglesUnits=deg  RotationMatrix=[1 0 0; 0 1 0; 0 0 1]  Quaternion=[1 0 0 0]  TranslationMethod=None  TranslationCartesianOffset=[0 0 0]  TranslationCartesianOffsetUnits=m  TranslationStandardAxis=+Z  TranslationStandardOffset=0  TranslationStandardOffsetUnits=m  TranslationROffset=0  TranslationROffsetUnits=m  TranslationThetaOffset=0  TranslationThetaOffsetUnits=deg  TranslationZOffset=0  TranslationZOffsetUnits=m
  Transform Revolute Z : sm_lib/Frames and Transforms/Rigid Transform  RotationMethod=AlignedAxes  FollAlignAxisA=+Y  BaseAlignAxisA=+Z  FollAlignAxisB=+X  BaseAlignAxisB=+X  RotationStandardAxis=+Z  RotationAngle=0.0  RotationAngleUnits=deg  RotationArbitraryAxis=[0 0 1]  RotationSequenceAxes=FollowerAxes  RotationSequence=XYX  RotationSequenceAngles=[0 0 0]  RotationSequenceAnglesUnits=deg  RotationMatrix=[1 0 0; 0 1 0; 0 0 1]  Quaternion=[1 0 0 0]  TranslationMethod=None  TranslationCartesianOffset=[0 0 0]  TranslationCartesianOffsetUnits=m  TranslationStandardAxis=+Z  TranslationStandardOffset=0  TranslationStandardOffsetUnits=m  TranslationROffset=0  TranslationROffsetUnits=m  TranslationThetaOffset=0  TranslationThetaOffsetUnits=deg  TranslationZOffset=0  TranslationZOffsetUnits=m
  B : PMIOPort  Side=Left
  F : PMIOPort  Port=2  Side=Right
  connections:
  B/RConn1 -- Transform Revolute X/LConn1
  Transform Revolute Z/RConn1 -- Revolute Z/LConn1
  Transform Revolute Y/RConn1 -- Revolute Y/LConn1
  Transform Revolute X/RConn1 -- Revolute X/LConn1
  Transform Revolute Z/LConn1 -- Revolute Y/RConn1
  F/RConn1 -- Revolute Z/RConn1
  Transform Revolute Y/LConn1 -- Revolute X/RConn1

== system MultibodySuspensionSSC/SuspR/Linkage/Linkage L/DoubleWishbone/Revolute LA ==
  Revolute LAc : sm_lib/Joints/Revolute Joint  JointMode=Normal  CompositeWrenchDir=FollowerOnBase  CompositeWrenchFrame=BaseFrame  SenseConstraintForce=off  SenseConstraintTorque=off  SenseTotalForce=off  SenseTotalTorque=off  PositionTargetSpecify=on  PositionTargetPriority=Low  PositionTargetValue=0  PositionTargetValueUnits=deg  VelocityTargetSpecify=off  VelocityTargetPriority=High  VelocityTargetValue=0  VelocityTargetValueUnits=deg/s  EquilibriumPosition=0  EquilibriumPositionUnits=deg  SpringStiffness=0  SpringStiffnessUnits=N*m/deg  DampingCoefficient=0.01  DampingCoefficientUnits=N*m/(deg/s)  LowerLimitSpecify=off  LowerLimitBound=-90  LowerLimitBoundUnits=deg  LowerLimitStiffness=1e4  LowerLimitStiffnessUnits=N*m/deg  LowerLimitDamping=10  LowerLimitDampingUnits=N*m/(deg/s)  LowerLimitTransitionRegionWidth=0.1  LowerLimitTransitionRegionWidthUnits=deg  UpperLimitSpecify=off  UpperLimitBound=90  UpperLimitBoundUnits=deg  UpperLimitStiffness=1e4  UpperLimitStiffnessUnits=N*m/deg  UpperLimitDamping=10  UpperLimitDampingUnits=N*m/(deg/s)  UpperLimitTransitionRegionWidth=0.1  UpperLimitTransitionRegionWidthUnits=deg  TorqueActuationMode=NoTorque  MotionActuationMode=ComputedMotion  SensePosition=off  SenseVelocity=off  SenseAcceleration=off  SenseTorqueForce=off  SenseLowerLimitTorqueForce=off  SenseUpperLimitTorqueForce=off
      settings: LibrarySourceBlock=sm_car_4post_lib/Suspension and Steering/Linkage/Linkage L/DoubleWishbone/Revolute LA/Revolute LAc
  Simscape Bus LA : SimscapeBus  HierarchyStrings=LAf;LAc;LAr
  Simscape Bus LA HP : SimscapeBus  HierarchyStrings=LAf;LAc;LAr
  Terminator LAf Chassis : Subsystem
      settings: LibrarySourceBlock=|
      | sm_car_4post_lib/Suspension and Steering/Linkage/Linkage L/DoubleWishbone/Revolute LA/Terminator
      | LAf Chassis
  Terminator LAf Susp : Subsystem
      settings: LibrarySourceBlock=|
      | sm_car_4post_lib/Suspension and Steering/Linkage/Linkage L/DoubleWishbone/Revolute LA/Terminator
      | LAf Susp
  Terminator LAr Chassis : Subsystem
      settings: LibrarySourceBlock=|
      | sm_car_4post_lib/Suspension and Steering/Linkage/Linkage L/DoubleWishbone/Revolute LA/Terminator
      | LAr Chassis
  Terminator LAr Susp : Subsystem
      settings: LibrarySourceBlock=|
      | sm_car_4post_lib/Suspension and Steering/Linkage/Linkage L/DoubleWishbone/Revolute LA/Terminator
      | LAr Susp
  F : PMIOPort  Side=Right
  B : PMIOPort  Port=2  Side=Left
  connections:
  Terminator LAr Susp/RConn1 -- Simscape Bus LA/LConn3
  Terminator LAr Chassis/RConn1 -- Simscape Bus LA HP/LConn3
  Terminator LAf Susp/RConn1 -- Simscape Bus LA/LConn1
  Terminator LAf Chassis/RConn1 -- Simscape Bus LA HP/LConn1
  Simscape Bus LA/RConn1 -- F/RConn1
  Revolute LAc/RConn1 -- Simscape Bus LA/LConn2
  Simscape Bus LA HP/LConn2 -- Revolute LAc/LConn1
  Simscape Bus LA HP/RConn1 -- B/RConn1

== system MultibodySuspensionSSC/SuspR/Linkage/Linkage L/DoubleWishbone/Revolute UA ==
  Revolute UAc : sm_lib/Joints/Revolute Joint  JointMode=Normal  CompositeWrenchDir=FollowerOnBase  CompositeWrenchFrame=BaseFrame  SenseConstraintForce=off  SenseConstraintTorque=off  SenseTotalForce=off  SenseTotalTorque=off  PositionTargetSpecify=on  PositionTargetPriority=Low  PositionTargetValue=0  PositionTargetValueUnits=deg  VelocityTargetSpecify=off  VelocityTargetPriority=High  VelocityTargetValue=0  VelocityTargetValueUnits=deg/s  EquilibriumPosition=0  EquilibriumPositionUnits=deg  SpringStiffness=0  SpringStiffnessUnits=N*m/deg  DampingCoefficient=0  DampingCoefficientUnits=N*m/(deg/s)  LowerLimitSpecify=off  LowerLimitBound=-90  LowerLimitBoundUnits=deg  LowerLimitStiffness=1e4  LowerLimitStiffnessUnits=N*m/deg  LowerLimitDamping=10  LowerLimitDampingUnits=N*m/(deg/s)  LowerLimitTransitionRegionWidth=0.1  LowerLimitTransitionRegionWidthUnits=deg  UpperLimitSpecify=off  UpperLimitBound=90  UpperLimitBoundUnits=deg  UpperLimitStiffness=1e4  UpperLimitStiffnessUnits=N*m/deg  UpperLimitDamping=10  UpperLimitDampingUnits=N*m/(deg/s)  UpperLimitTransitionRegionWidth=0.1  UpperLimitTransitionRegionWidthUnits=deg  TorqueActuationMode=NoTorque  MotionActuationMode=ComputedMotion  SensePosition=off  SenseVelocity=off  SenseAcceleration=off  SenseTorqueForce=off  SenseLowerLimitTorqueForce=off  SenseUpperLimitTorqueForce=off
      settings: LibrarySourceBlock=sm_car_4post_lib/Suspension and Steering/Linkage/Linkage L/DoubleWishbone/Revolute UA/Revolute UAc
  Simscape Bus : SimscapeBus  HierarchyStrings=UAf;UAc;UAr
  Simscape Bus1 : SimscapeBus  HierarchyStrings=UAf;UAc;UAr
  Terminator UAf Chassis : Subsystem
      settings: LibrarySourceBlock=|
      | sm_car_4post_lib/Suspension and Steering/Linkage/Linkage L/DoubleWishbone/Revolute UA/Terminator
      | UAf Chassis
  Terminator UAf Susp : Subsystem
      settings: LibrarySourceBlock=|
      | sm_car_4post_lib/Suspension and Steering/Linkage/Linkage L/DoubleWishbone/Revolute UA/Terminator
      | UAf Susp
  Terminator UAr Chassis : Subsystem
      settings: LibrarySourceBlock=|
      | sm_car_4post_lib/Suspension and Steering/Linkage/Linkage L/DoubleWishbone/Revolute UA/Terminator
      | UAr Chassis
  Terminator UAr Susp : Subsystem
      settings: LibrarySourceBlock=|
      | sm_car_4post_lib/Suspension and Steering/Linkage/Linkage L/DoubleWishbone/Revolute UA/Terminator
      | UAr Susp
  F : PMIOPort  Side=Right
  " B" : PMIOPort  Port=2  Side=Left
  connections:
  Terminator UAr Chassis/RConn1 -- Simscape Bus/LConn3
  Terminator UAf Chassis/RConn1 -- Simscape Bus/LConn1
  Terminator UAr Susp/RConn1 -- Simscape Bus1/LConn3
  Terminator UAf Susp/RConn1 -- Simscape Bus1/LConn1
  Simscape Bus1/RConn1 -- F/RConn1
  Simscape Bus/RConn1 -- " B"/RConn1
  Simscape Bus1/LConn2 -- Revolute UAc/RConn1
  Simscape Bus/LConn2 -- Revolute UAc/LConn1

== system MultibodySuspensionSSC/SuspR/Linkage/Linkage L/DoubleWishbone/Shock ==
  Cylinder : Subsystem
  MTRef : fl_lib/Mechanical/Translational Elements/Mechanical Translational Reference
      settings: LibrarySourceBlock=sm_car_4post_lib/Suspension and Steering/Linkage/Linkage L/DoubleWishbone/Shock/MTRef
  Piston : Subsystem
  Prismatic Spring : sm_lib/Joints/Prismatic Joint  JointMode=Normal  CompositeWrenchDir=FollowerOnBase  CompositeWrenchFrame=BaseFrame  SenseConstraintForce=off  SenseConstraintTorque=off  SenseTotalForce=off  SenseTotalTorque=off  PositionTargetSpecify=on  PositionTargetPriority=High  PositionTargetValue=init_spr_len  PositionTargetValueUnits=m  VelocityTargetSpecify=off  VelocityTargetPriority=High  VelocityTargetValue=0  VelocityTargetValueUnits=m/s  EquilibriumPosition=0  EquilibriumPositionUnits=m  SpringStiffness=0  SpringStiffnessUnits=N/m  DampingCoefficient=0  DampingCoefficientUnits=N/(m/s)  LowerLimitSpecify=off  LowerLimitBound=-1  LowerLimitBoundUnits=m  LowerLimitStiffness=1e6  LowerLimitStiffnessUnits=N/m  LowerLimitDamping=1e3  LowerLimitDampingUnits=N/(m/s)  LowerLimitTransitionRegionWidth=1e-4  LowerLimitTransitionRegionWidthUnits=m  UpperLimitSpecify=off  UpperLimitBound=1  UpperLimitBoundUnits=m  UpperLimitStiffness=1e6  UpperLimitStiffnessUnits=N/m  UpperLimitDamping=1e3  UpperLimitDampingUnits=N/(m/s)  UpperLimitTransitionRegionWidth=1e-4  UpperLimitTransitionRegionWidthUnits=m  TorqueActuationMode=InputTorque  MotionActuationMode=ComputedMotion  SensePosition=off  SenseVelocity=on  SenseAcceleration=off  SenseTorqueForce=off  SenseLowerLimitTorqueForce=off  SenseUpperLimitTorqueForce=off
      settings: LibrarySourceBlock=|
      | sm_car_4post_lib/Suspension and Steering/Linkage/Linkage L/DoubleWishbone/Shock/Prismatic
      | Spring
  Translational Multibody Interface : fl_lib/Mechanical/Multibody Interfaces/Translational Multibody Interface
      settings: LibrarySourceBlock=|
      | sm_car_4post_lib/Suspension and Steering/Linkage/Linkage L/DoubleWishbone/Shock/Translational
      | Multibody Interface
  Vis Spring HP : sm_lib/Body Elements/Spherical Solid  SphereRadius=size_conn_shock  SphereRadiusUnits=m  ExportEntireGeometry=off  InertiaType=PointMass  BasedOnType=Density  Density=0  DensityUnits=kg/m^3  Mass=0  MassUnits=kg  CenterOfMass=[0 0 0]  CenterOfMassUnits=m  MomentsOfInertia=[1 1 1]  MomentsOfInertiaUnits=kg*m^2  ProductsOfInertia=[0 0 0]  ProductsOfInertiaUnits=kg*m^2  GraphicType=FromGeometry  MarkerShape=Sphere  MarkerSize=10  GraphicVisPropType=SimpleVisualProperties  GraphicDiffuseColor=clr_conn_shock  GraphicOpacity=opc_conn_shock  GraphicSpecularColor=[0.5 0.5 0.5 1.0]  GraphicAmbientColor=[0.15 0.15 0.15 1.0]  GraphicEmissiveColor=[0.0 0.0 0.0 1.0]  GraphicShininess=75  DoExposeReferenceFrame=on  SerializedFrames=<Frames/>
      settings: LibrarySourceBlock=|
      | sm_car_4post_lib/Suspension and Steering/Linkage/Linkage L/DoubleWishbone/Shock/Vis
      | Spring
      | HP
  Vis Spring LA : sm_lib/Body Elements/Spherical Solid  SphereRadius=size_conn_shock  SphereRadiusUnits=m  ExportEntireGeometry=off  InertiaType=PointMass  BasedOnType=Density  Density=0  DensityUnits=kg/m^3  Mass=0  MassUnits=kg  CenterOfMass=[0 0 0]  CenterOfMassUnits=m  MomentsOfInertia=[1 1 1]  MomentsOfInertiaUnits=kg*m^2  ProductsOfInertia=[0 0 0]  ProductsOfInertiaUnits=kg*m^2  GraphicType=FromGeometry  MarkerShape=Sphere  MarkerSize=10  GraphicVisPropType=SimpleVisualProperties  GraphicDiffuseColor=clr_conn_shock  GraphicOpacity=opc_conn_shock  GraphicSpecularColor=[0.5 0.5 0.5 1.0]  GraphicAmbientColor=[0.15 0.15 0.15 1.0]  GraphicEmissiveColor=[0.0 0.0 0.0 1.0]  GraphicShininess=75  DoExposeReferenceFrame=on  SerializedFrames=<Frames/>
      settings: LibrarySourceBlock=|
      | sm_car_4post_lib/Suspension and Steering/Linkage/Linkage L/DoubleWishbone/Shock/Vis
      | Spring
      | LA
  R : PMIOPort  Side=Right
  HP : PMIOPort  Port=2  Side=Right
  LA : PMIOPort  Port=3  Side=Left
  connections:
  Translational Multibody Interface/RConn2 -- R/RConn1
  Translational Multibody Interface/LConn2 -- MTRef/LConn1
  HP/RConn1 -- Piston/RConn1 -- Prismatic Spring/RConn1 -- Vis Spring HP/RConn1
  Prismatic Spring/LConn1 -- Cylinder/LConn1 -- LA/RConn1 -- Vis Spring LA/RConn1
  Translational Multibody Interface/RConn1 -- Prismatic Spring/RConn2
  Prismatic Spring/LConn2 -- Translational Multibody Interface/LConn1
